simulink model "stateflow_demo_adding_ports"  (R2014a)
settings: Solver=FixedStepDiscrete  StartTime=0.0  StopTime=10.0  RelTol=1e-3
settings Model: Creator=mprior  LastModifiedBy=mprior
settings DataIOCC: LimitDataPoints=off  SaveOutput=off  SaveTime=off
settings DebuggingCC: SolverPrmCheckMsg=none  SingleTaskRateTransMsg=error

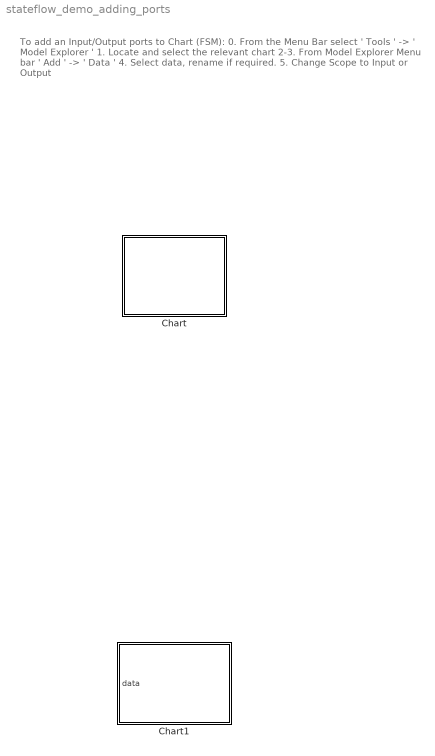
== system stateflow_demo_adding_ports ==
  note: To add an Input/Output ports to Chart (FSM):
      | 0. From the Menu Bar select ' Tools ' -> ' Model Explorer '
      | 1. Locate and select the relevant chart
      | 2-3. From Model Explorer Menu bar ' Add ' -> ' Data '
      | 4. Select data, rename if required.
      | 5. Change Scope to Input or Output
  Chart : Stateflow chart  TreatAsAtomicUnit=on
  Chart1 : Stateflow chart  TreatAsAtomicUnit=on

== stateflow chart stateflow_demo_adding_ports/Chart1 ==
  data: data input

== stateflow chart stateflow_demo_adding_ports/Chart ==
